simulink model "simTP1_2020a"  (R2024b)
settings: Solver=ode1  StartTime=0.0  StopTime=9  FixedStep=1e-5  RelTol=1e-9
values from neighbouring files (symbols this model uses):
  Delta = 4    [scriptTP1.m]
  dVtheta_dt0 = 0    [scriptTP1.m]
  k2 = 0    [scriptTP1.m]
  Kg = 0.0129    [scriptTP1.m]
  Km = 38.57    [scriptTP1.m]
  Ks = 1.57    [scriptTP1.m]
  M = 6    [scriptTP1.m]
  tau = 0.27    [scriptTP1.m]
  Vtheta0 = dVtheta_dt0 =      simOut = sim('simTP1_2023a.slx')    [scriptTP1.m]
settings Model: Creator=yariba  LastModifiedBy=yariba
settings RTWCC: GPUComputeCapability=3.5

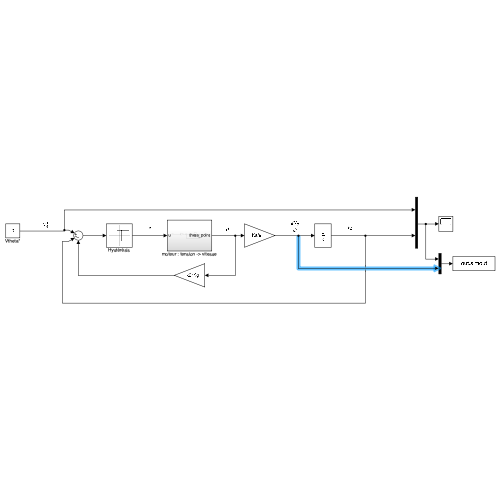
[thumbnail: Simulink's stored preview of the top-level diagram]
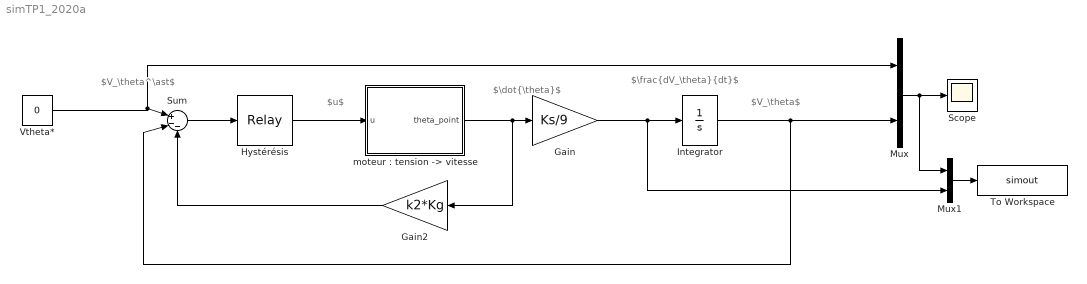
== system simTP1_2020a ==
  note: $u$
  note: $V_\theta$
  note: $\frac{dV_\theta}{dt}$
  note: $\dot{\theta}$
  note: $V_\theta^\ast$
  Gain : Gain  Gain=Ks/9
  Gain2 : Gain  Gain=k2*Kg
  Hystérésis : Relay  OnSwitchValue=Delta/2  OffSwitchValue=-Delta/2  OnOutputValue=M  OffOutputValue=-M
  Integrator : Integrator  InitialCondition=Vtheta0
  Mux : Mux  Inputs=2
  Mux1 : Mux  Inputs=2
  Scope : Scope
  Sum : Sum  Inputs=|+--
  To Workspace : ToWorkspace  VariableName=simout  SaveFormat=Timeseries  SampleTime=-1
  Vtheta* : Constant  Value=0
  "moteur : tension -> vitesse" : Subsystem
  wires:
  Gain/1 -> Mux1/2, Integrator/1
  "moteur : tension -> vitesse"/1(theta_point) -> Gain2/1, Gain/1
  Hystérésis/1 -> "moteur : tension -> vitesse"/1(u)
  Sum/1 -> Hystérésis/1
  Integrator/1 -> Sum/2, Mux/2
  Mux/1 -> Mux1/1, Scope/1
  Vtheta*/1 -> Mux/1, Sum/1
  Gain2/1 -> Sum/3
  Mux1/1 -> To Workspace/1

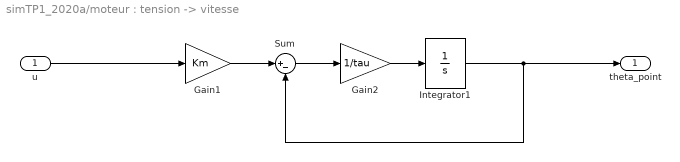
== system simTP1_2020a/moteur : tension -> vitesse ==
  u : Inport
  Gain1 : Gain  Gain=Km
  Gain2 : Gain  Gain=1/tau
  Integrator1 : Integrator  InitialCondition=dVtheta_dt0*9/Ks
  Sum : Sum  Inputs=|+-
  theta_point : Outport
  wires:
  u/1 -> Gain1/1
  Gain1/1 -> Sum/1
  Sum/1 -> Gain2/1
  Gain2/1 -> Integrator1/1
  Integrator1/1 -> theta_point/1, Sum/2
